simulink subsystem "RT_BladePitchAngles_v1_2"  (R2025a)
settings: Solver=VariableStepAuto  StartTime=0.0  StopTime=10.0  RelTol=1e-3
settings Model: DefaultTestHarness=RT_BladePitchAngles_v1_1_Harness1  Creator=Admin  LastModifiedBy=Admin

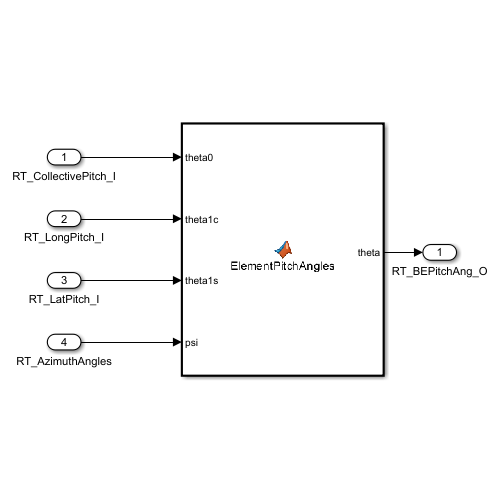
[thumbnail: Simulink's stored preview of the top-level diagram]
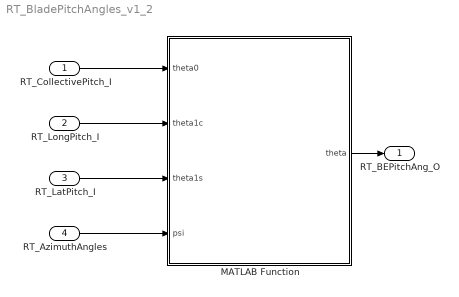
== system RT_BladePitchAngles_v1_2 ==
  RT_CollectivePitch_I : Inport
  RT_LongPitch_I : Inport  Port=2
  RT_LatPitch_I : Inport  Port=3
  RT_AzimuthAngles : Inport  Port=4
  MATLAB Function : MATLAB Function  TreatAsAtomicUnit=on
  RT_BEPitchAng_O : Outport
  wires:
  RT_CollectivePitch_I/1 -> MATLAB Function/1(theta0)
  RT_LongPitch_I/1 -> MATLAB Function/2(theta1c)
  RT_LatPitch_I/1 -> MATLAB Function/3(theta1s)
  RT_AzimuthAngles/1 -> MATLAB Function/4(psi)
  MATLAB Function/1(theta) -> RT_BEPitchAng_O/1

== matlab function RT_BladePitchAngles_v1_2/MATLAB Function ==
  data: theta0 input; theta output; theta1c input; theta1s input; psi input
function theta = ElementPitchAngles(theta0,theta1c,theta1s,psi)

theta = ones(4,20).*(theta0+theta1c*cos(psi)+theta1s*sin(psi));
